simulink model "ADCModel_control101"  (R2024a)
settings: Solver=VariableStepAuto  StartTime=0.0  StopTime=StopTime  FixedStep=0.1  RelTol=1e-3
undefined symbols (not defined in the file or in its folder): ProjectLib, resolution, SampleTime, Saturation, sensormax, sensormin
settings Model: Creator=sword  LastModifiedBy=Anthony Rossiter
settings RTWCC: GPUComputeCapability=3.5
settings ConfigComp: CovBoundaryAbsTol=1.0e-5

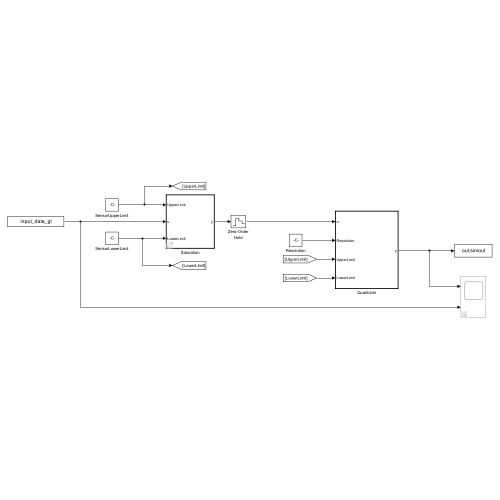
[thumbnail: Simulink's stored preview of the top-level diagram]
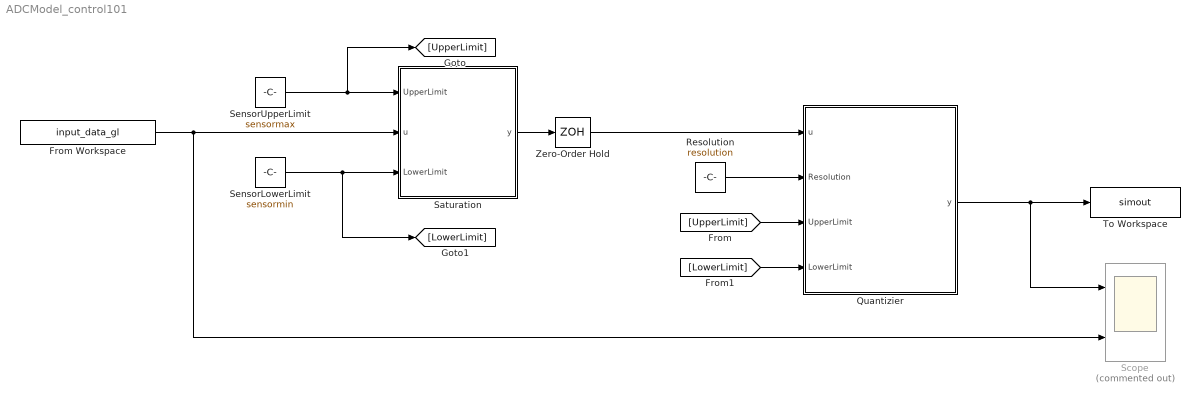
== system ADCModel_control101 ==
  From Workspace : FromWorkspace  VariableName=input_data_gl  SampleTime=0.0001
  Quantizier : Subsystem  TreatAsAtomicUnit=on
      settings: RTWSystemCode=Inline
  Resolution : Constant  Value=resolution  SampleTime=-1
  Saturation : Subsystem  AncestorBlock=ProjectLib/Saturation  TreatAsAtomicUnit=on
      settings: RTWSystemCode=Inline
  Scope : Scope  Commented=on  NumInputPorts=2
  SensorLowerLimit : Constant  Value=sensormin  SampleTime=-1
  SensorUpperLimit : Constant  Value=sensormax  SampleTime=-1
  To Workspace : ToWorkspace  VariableName=simout  SaveFormat=Structure With Time  SampleTime=SampleTime
  Zero-Order Hold : ZeroOrderHold  SampleTime=0.1
  wires:
  SensorUpperLimit/1 -> [UpperLimit], Saturation/1(UpperLimit)
  SensorLowerLimit/1 -> [LowerLimit], Saturation/3(LowerLimit)
  Saturation/1(y) -> Zero-Order Hold/1
  From Workspace/1 -> Scope/2, Saturation/2(u)
  Quantizier/1(y) -> To Workspace/1, Scope/1
  [UpperLimit] -> Quantizier/3(UpperLimit)
  [LowerLimit] -> Quantizier/4(LowerLimit)
  Resolution/1 -> Quantizier/2(Resolution)
  Zero-Order Hold/1 -> Quantizier/1(u)

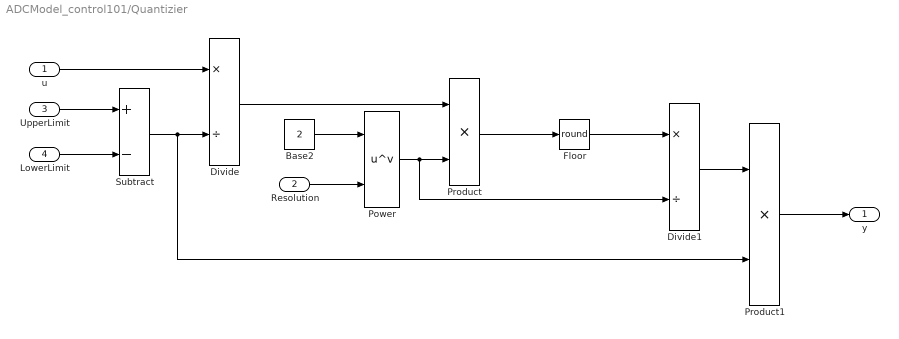
== system ADCModel_control101/Quantizier ==
  u : Inport
  Resolution : Inport  Port=2
  UpperLimit : Inport  Port=3
  LowerLimit : Inport  Port=4
  Base2 : Constant  Value=2  SampleTime=-1
  Divide : Product  Inputs=*/
  Divide1 : Product  Inputs=*/
  Floor : Rounding  Operator=round
  Power : Math  Operator=pow
  Product : Product
  Product1 : Product
  Subtract : Sum  Inputs=+-
  y : Outport
  wires:
  Divide1/1 -> Product1/1
  Subtract/1 -> Product1/2, Divide/2
  Floor/1 -> Divide1/1
  UpperLimit/1 -> Subtract/1
  Product/1 -> Floor/1
  Power/1 -> Product/2, Divide1/2
  Product1/1 -> y/1
  Base2/1 -> Power/1
  LowerLimit/1 -> Subtract/2
  Resolution/1 -> Power/2
  Divide/1 -> Product/1
  u/1 -> Divide/1

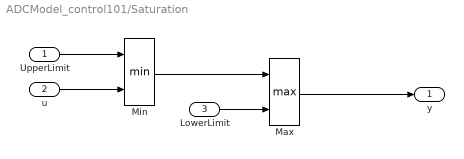
== system ADCModel_control101/Saturation ==
  UpperLimit : Inport
  u : Inport  Port=2
  LowerLimit : Inport  Port=3
  Max : MinMax  Function=max  Inputs=2
  Min : MinMax  Inputs=2
  y : Outport
  wires:
  LowerLimit/1 -> Max/2
  u/1 -> Min/2
  UpperLimit/1 -> Min/1
  Min/1 -> Max/1
  Max/1 -> y/1
